simulink model "LotkaVolterra"  (R2020a)
settings: Solver=ode23  StartTime=0.0  StopTime=100  RelTol=1e-3
values from neighbouring files (symbols this model uses):
  alpha = 0.02    [main.m]
  beta = 0.01    [main.m]
  x0 = 20    [main.m]
  y0 = 10    [main.m]
settings Model: Creator=tulpule.3  LastModifiedBy=tulpule.3

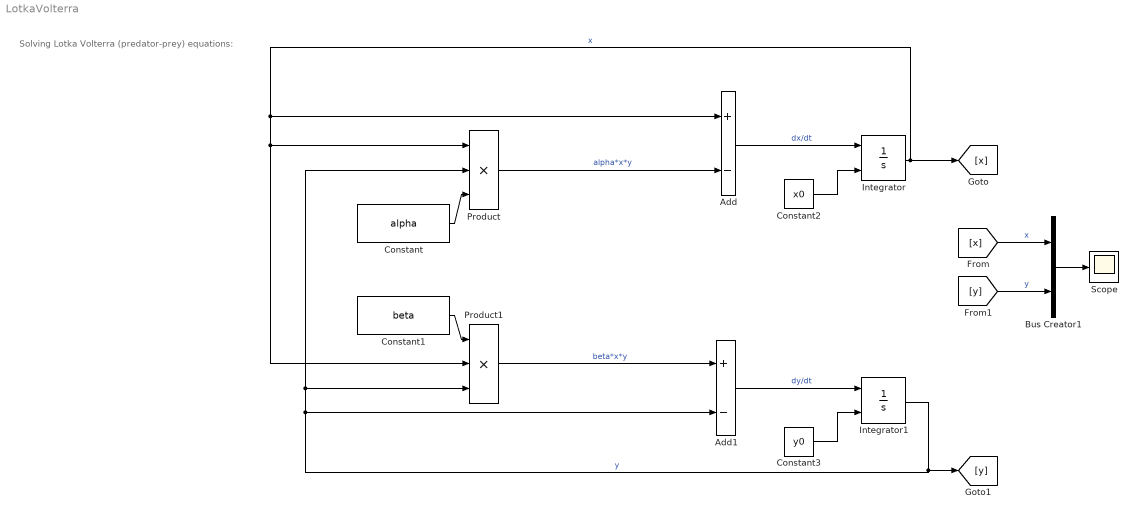
== system LotkaVolterra ==
  note: Solving Lotka Volterra (predator-prey) equations:
  Add : Sum  Inputs=+-
  Add1 : Sum  Inputs=+-
  Bus Creator1 : BusCreator  Inputs=2
  Constant : Constant  Value=alpha
  Constant1 : Constant  Value=beta
  Constant2 : Constant  Value=x0
  Constant3 : Constant  Value=y0
  Integrator : Integrator  InitialConditionSource=external
  Integrator1 : Integrator  InitialConditionSource=external
  Product : Product  Inputs=3
  Product1 : Product  Inputs=3
  Scope : Scope
  wires:
  Integrator/1 -> [x], Product1/2, Product/1, Add/1  "x"
  Integrator1/1 -> Product/2, Product1/3, Add1/2, [y]  "y"
  Constant/1 -> Product/3
  Product/1 -> Add/2  "alpha*x*y"
  Add/1 -> Integrator/1  "dx/dt"
  Constant1/1 -> Product1/1
  Product1/1 -> Add1/1  "beta*x*y"
  Add1/1 -> Integrator1/1  "dy/dt"
  Constant2/1 -> Integrator/2
  Constant3/1 -> Integrator1/2
  [y] -> Bus Creator1/2  "y"
  [x] -> Bus Creator1/1  "x"
  Bus Creator1/1 -> Scope/1
